simulink library "solarpvmodel"  (R2019a)
settings: Solver=VariableStepAuto  StartTime=0.0  StopTime=10.0  RelTol=1e-3
undefined symbols (not defined in the file): Acid, Lead
libraries: powerlib x7, electricdrivelib x1, re_lib x1, powerlib_meascontrol x1
settings Model: Creator=Adnan Computers  LastModifiedBy=Adnan Computers

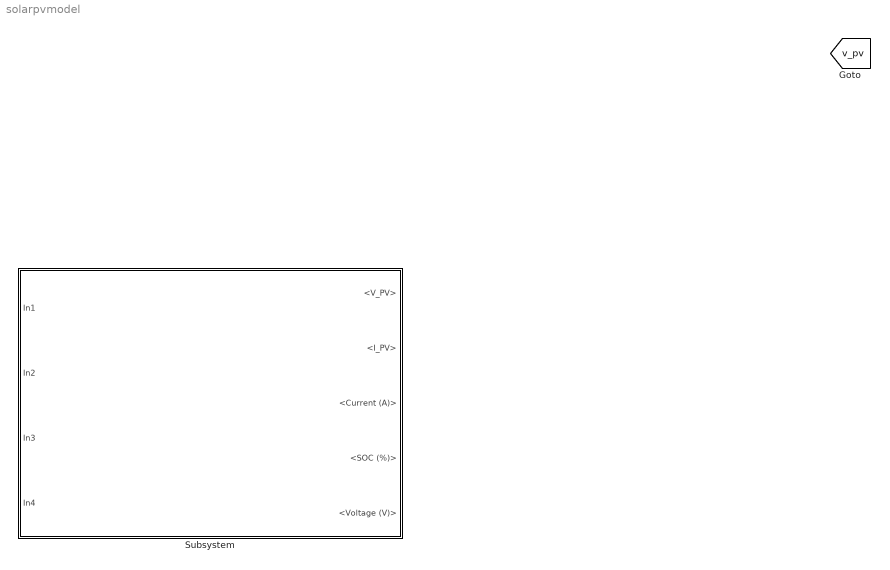
== system solarpvmodel ==
  Subsystem : Subsystem
  tag scope: v_pv=global
  wires:
  ? -> ?

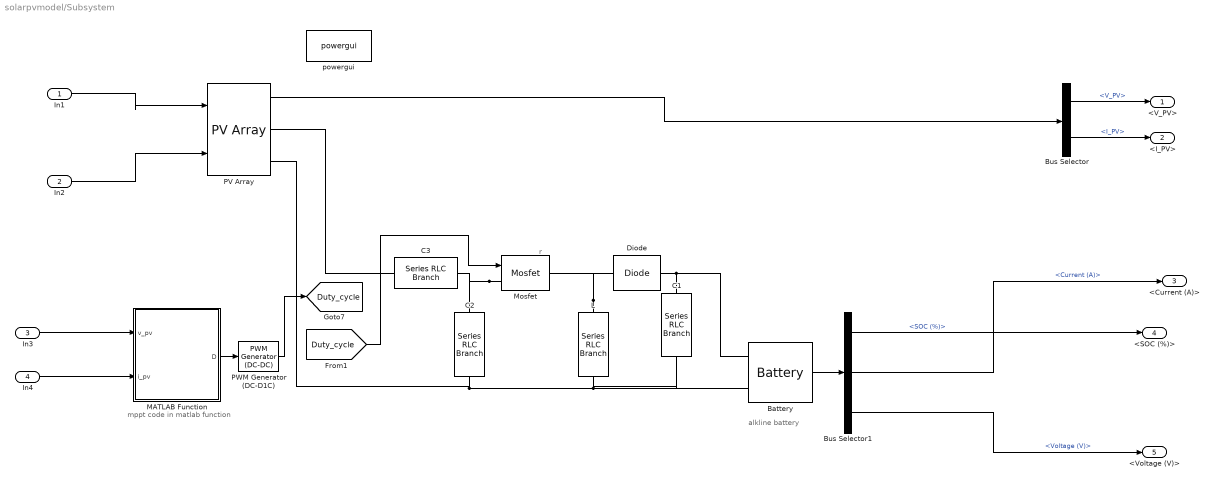
== system solarpvmodel/Subsystem ==
  note: alkline battery
  note: mppt code in matlab function
  note: r
  In1 : Inport
  In2 : Inport  Port=2
  In3 : Inport  Port=3
  In4 : Inport  Port=4
  Battery : electricdrivelib/Extra Sources/Battery  BatType=Lead-Acid  ShowTempParam=off  ThermalPreset=no  ShowAgeParam=off  NomV=12  NomQ=100  SOC=45  Batt_Tr=1  PresetModel=on  MaxQ=104.1667  MinV=9  FullV=13.0658  Dis_rate=20  R=0.0012  Normal_OP=31.0278  expZone="[12.2171     0.333333]"  current=[6.5 13 32.5]  Units=Time  Tci=20  NomT=20  T2=-30  MaxQ2=4.8  FullV2=7.1  Normal_OP2=5.655  expZone2="[6.58           1]"  Rca=0.6  ti=2000  Dp=0  Neq0=0  Tsim=1e6  Ta1=25  Qeol=5.4*0.9  Reol=0.013333*1.2  Char_age=[2.3478, 3]  Dis_age=[2.3478, 10]  N1=1500  N2=10500  N3=1000  N4=1400  Ta2=45  N5=950
      settings: SourceProductName=Simscape Electrical
  Bus Selector : BusSelector  OutputSignals=V_PV,I_PV
  Bus Selector1 : BusSelector  OutputSignals=SOC (%),Current (A),Voltage (V)
  C1 : powerlib/Elements/Series RLC Branch  LConnTagsString=__new0  RConnTagsString=__new0  BranchType=C  Resistance=1  Inductance=1e-3  SetiL0=off  InitialCurrent=0  Capacitance=1.850e-6  Setx0=off  InitialVoltage=0  Measurements=None
      settings: SourceProductName=Simscape Electrical
  C2 : powerlib/Elements/Series RLC Branch  LConnTagsString=__new0  RConnTagsString=__new0  BranchType=C  Resistance=0.001  Inductance=1e-3  SetiL0=off  InitialCurrent=0  Capacitance=1000e-6  Setx0=off  InitialVoltage=0  Measurements=None
      settings: SourceProductName=Simscape Electrical
  C3 : powerlib/Elements/Series RLC Branch  LConnTagsString=__new0  RConnTagsString=__new0  BranchType=R  Resistance=0.0001  Inductance=1e-3  SetiL0=off  InitialCurrent=0  Capacitance=1000e-6  Setx0=off  InitialVoltage=0  Measurements=None
      settings: SourceProductName=Simscape Electrical
  Diode : powerlib/Power Electronics/Diode  Ron=0.001  Lon=0  Vf=0.8  IC=0  UseSnubber=0  Rs=500  Cs=250e-9  Measurements=off
      settings: SourceProductName=Simscape Electrical
  L : powerlib/Elements/Series RLC Branch  LConnTagsString=__new0  RConnTagsString=__new0  BranchType=L  Resistance=1  Inductance=1.92e-6  SetiL0=off  InitialCurrent=0  Capacitance=1e-6  Setx0=off  InitialVoltage=0  Measurements=None
      settings: SourceProductName=Simscape Electrical
  MATLAB Function : MATLAB Function  TreatAsAtomicUnit=on
  Mosfet : powerlib/Power Electronics/Mosfet  Ron=0.1  Lon=0  Rd=0.01  Vfd=0  IC=0  Rs=1e5  Cs=inf  Measurements=off
      settings: SourceProductName=Simscape Electrical
  PV Array : re_lib/Solar/PV Array  Npar=1  Nser=1  PlotType=one module @ 25 deg.C & specified irradiances  S_vec="[ 1000  500  100 ]"  Temp_C_vec="[ 45 25  ]"  ModuleName=User-defined  PlotWhenSelected=off  Pm=213.15  Ncell=60  Voc=36.3  Isc=7.84  Vm=29  Im=7.35  beta_Voc_pc=-0.36099  alpha_Isc_pc=0.102  beta_Voc=-0.13104  alpha_Isc=0.0079968  IL=7.8654  I0=2.9273e-10  nI=0.98119  Rsh=313.0553  Rs=0.39381  BAL=on  Tc=1e-6  Tfilter=5e-5
      settings: SourceProductName=Simscape Electrical
  PWM Generator (DC-D1C) : powerlib_meascontrol/Pulse & Signal Generators/PWM Generator (DC-DC)  Fsw=25000  Ts=10e-6
      settings: SourceProductName=Simscape Electrical
  powergui : powerlib/powergui  Priority=1  SimulationMode=Discrete  SampleTime=10e-6  frequency=60  Iterations=50  frequencyindice=0  Pbase=100e6  ErrMax=1e-4  UnitsV=kV  UnitsW=MW  buscounter=0  FunctionMessages=off  echomessages=off  EnableUseOfTLC=off  CurrentSourceSwitches=off  DisableSnubberDevices=off  DisableRonSwitches=off  DisableVfSwitches=off  DisplayEquations=off  AutomaticDiscreteSolvers=off  SolverType=Tustin/Backward Euler (TBE)  Interpol=off  ExternalGateDelay=off  methode=off  Ts=100  x0status=blocks  SPID=on  SwTol=0  HookPort=off  NonlinearTolerance=1e-4  nMaxIteration=100  ContinueOnMaxIteration=off  RestoreLinks=warning  ResistiveCurrentMeasurement=off  Frange=[0:2:500]  Ylog=off  Xlog=on  ShowGrid=off  save=off  variable=ZData  structure=0  ZoomFFT=off  StartTime=0.0  cycles=1  DisplayStyle=1  fundamental=60  FreqAxis=off  MaxFrequency=1000  frequencyindicesteady=1  RmsSteady=1  display=off
      settings: SourceProductName=Simscape Electrical
  <V_PV> : Outport
  <I_PV> : Outport  Port=2
  <Current (A)> : Outport  Port=3
  <SOC (%)> : Outport  Port=4
  <Voltage (V)> : Outport  Port=5
  tag scope: Duty_cycle=global
  wires:
  [Duty_cycle] -> Mosfet/1
  Bus Selector/2 -> <I_PV>/1  "<I_PV>"
  PV Array/1 -> Bus Selector/1
  Battery/1 -> Bus Selector1/1
  PWM Generator (DC-D1C)/1 -> [Duty_cycle]
  MATLAB Function/1(D) -> PWM Generator (DC-D1C)/1
  Bus Selector1/2 -> <Current (A)>/1  "<Current (A)>"
  In1/1 -> PV Array/1
  Bus Selector1/3 -> <Voltage (V)>/1  "<Voltage (V)>"
  In3/1 -> MATLAB Function/1(v_pv)
  Bus Selector/1 -> <V_PV>/1  "<V_PV>"
  Bus Selector1/1 -> <SOC (%)>/1  "<SOC (%)>"
  In4/1 -> MATLAB Function/2(i_pv)
  In2/1 -> PV Array/2
  connections:
  L/LConn1 -- Mosfet/RConn1 -- Diode/RConn1
  C2/RConn1 -- PV Array/RConn2 -- Battery/LConn1 -- C1/RConn1 -- L/RConn1
  C1/LConn1 -- Battery/LConn2 -- Diode/LConn1
  C3/RConn1 -- PV Array/RConn1
  Mosfet/LConn1 -- C3/LConn1 -- C2/LConn1

== matlab function solarpvmodel/Subsystem/MATLAB Function ==
  data: v_pv input; D output; i_pv input
function D = pando(v_pv,i_pv)
persistent Dprev Pprev Vprev 
if isempty(Dprev)
    Dprev =0.6;
    Vprev = 35;
    Pprev =213;
end

deltaD=0.00004;
Ppv=v_pv*i_pv;

if (Ppv - Pprev )~=0
    if(Ppv - Pprev) > 0
        if (v_pv - Vprev) > 0
            D = Dprev - deltaD;
        else
            D = Dprev + deltaD;
        end
    else 
        if (v_pv - Vprev) > 0
            D = Dprev + deltaD;
        else
            D = Dprev - deltaD;
        end
    end
else 
    D = Dprev ;
end
Dprev = D ;
Pprev = Ppv ;
Vprev = v_pv ;
